simulink subsystem "manipulability_and_collinearity"  (R2022b)
settings: Solver=VariableStepAuto  StartTime=0.0  StopTime=10.0  RelTol=1e-3
settings Model: Creator=emu  LastModifiedBy=emu

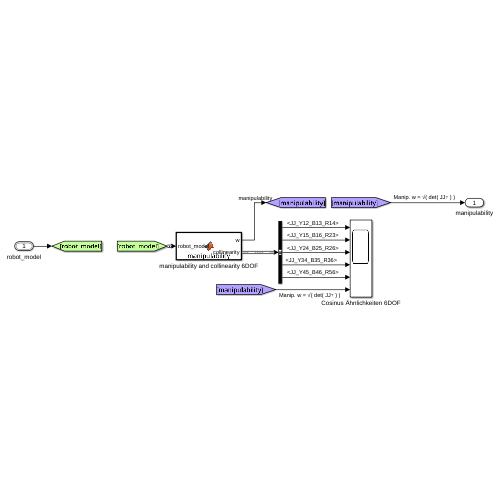
[thumbnail: Simulink's stored preview of the top-level diagram]
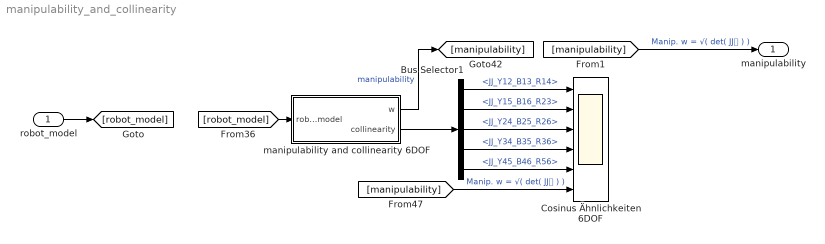
== system manipulability_and_collinearity ==
  robot_model : Inport  OutDataTypeStr=Bus: robot_model
  Bus Selector1 : BusSelector  OutputSignals=JJ_Y12_B13_R14,JJ_Y15_B16_R23,JJ_Y24_B25_R26,JJ_Y34_B35_R36,JJ_Y45_B46_R56
  Cosinus Ähnlichkeiten 6DOF : Scope  NumInputPorts=6
  manipulability and collinearity 6DOF : MATLAB Function  TreatAsAtomicUnit=on
  manipulability : Outport
  wires:
  [robot_model] -> manipulability and collinearity 6DOF/1(robot_model)
  [manipulability] -> Cosinus Ähnlichkeiten 6DOF/6  "Manip. w = √( det( JJ⸆ ) )"
  Bus Selector1/3 -> Cosinus Ähnlichkeiten 6DOF/3  "<JJ_Y24_B25_R26>"
  Bus Selector1/1 -> Cosinus Ähnlichkeiten 6DOF/1  "<JJ_Y12_B13_R14>"
  manipulability and collinearity 6DOF/2(collinearity) -> Bus Selector1/1
  Bus Selector1/5 -> Cosinus Ähnlichkeiten 6DOF/5  "<JJ_Y45_B46_R56>"
  manipulability and collinearity 6DOF/1(w) -> [manipulability]  "manipulability"
  Bus Selector1/2 -> Cosinus Ähnlichkeiten 6DOF/2  "<JJ_Y15_B16_R23>"
  Bus Selector1/4 -> Cosinus Ähnlichkeiten 6DOF/4  "<JJ_Y34_B35_R36>"
  robot_model/1 -> [robot_model]
  [manipulability] -> manipulability/1  "Manip. w = √( det( JJ⸆ ) )"

== matlab function manipulability_and_collinearity/manipulability and collinearity 6DOF ==
  settings: sampleTime=param_global.Ta
  data: robot_model input; w output; init_bus_param parameter; collinearity output Bus: collinearity_bus
function [w, collinearity]   = manipulability(robot_model, init_bus_param)

J = robot_model.J;
det_J = det(J*J');
w = sqrt(abs(det_J));

J_tilde = J./vecnorm(J);
JJ_colin = J_tilde'*J_tilde;

collinearity = init_bus_param.init_collinearity_bus;

% for 6 DOF CASE
collinearity.JJ_Y12_B13_R14 = [JJ_colin(1,2); JJ_colin(1,3); JJ_colin(1,4)]; 
collinearity.JJ_Y15_B16_R23 = [JJ_colin(1,5); JJ_colin(1,6); JJ_colin(2,3)];
collinearity.JJ_Y24_B25_R26 = [JJ_colin(2,4); JJ_colin(2,5); JJ_colin(2,6)];
collinearity.JJ_Y34_B35_R36 = [JJ_colin(3,4); JJ_colin(3,5); JJ_colin(3,6)];
collinearity.JJ_Y45_B46_R56 = [JJ_colin(4,5); JJ_colin(4,6); JJ_colin(5,6)];
